simulink model "es6"  (Simulink 8.1)
settings: Solver=ode45  StartTime=0.0  StopTime=10  RelTol=1e-3
libraries: cstblocks x4
settings Model: Creator=nessuno  LastModifiedBy=paolo
settings DataIOCC: SignalLoggingSaveFormat=Dataset
settings OptimizationCC: ExpressionDepthLimit=128
settings DebuggingCC: FcnCallInpInsideContextMsg=EnableAllAsError
settings GRTTargetCC: CombineOutputUpdateFcns=on  GRTInterface=off

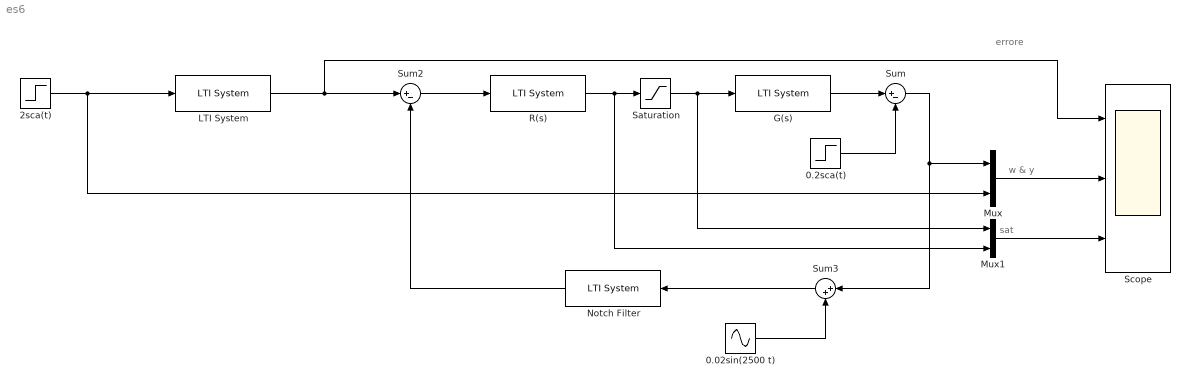
== system es6 ==
  note: sat
  note: w & y
  note: errore
  0.02sin(2500 t) : Sin  Amplitude=0.02  Frequency=2500  SampleTime=0
  0.2sca(t) : Step  Time=0  Before=1  After=0.2  SampleTime=0
  2sca(t) : Step  Time=2  After=2  SampleTime=0
  G(s) : cstblocks/LTI System  sys=G  IC=[]
  LTI System : cstblocks/LTI System  sys=PF  IC=[]
  Mux : Mux  Inputs=2
  Mux1 : Mux  Inputs=2
  Notch Filter : cstblocks/LTI System  sys=F_notch  IC=[]
  R(s) : cstblocks/LTI System  sys=R  IC=[]
  Saturation : Saturate  UpperLimit=2.39  LowerLimit=-0.24
  Scope : Scope  NumInputPorts=3
      settings: ShowLegends=on  TimeRange=10  YMin=-5~-5~-5  YMax=5~5~5
  Sum : Sum  Inputs=|+-
  Sum2 : Sum  Inputs=|+-
  Sum3 : Sum  Inputs=|++
  wires:
  Sum/1 -> Sum3/1, Mux/1
  LTI System/1 -> Sum2/1, Scope/1
  Sum2/1 -> R(s)/1
  G(s)/1 -> Sum/1
  R(s)/1 -> Mux1/2, Saturation/1
  Saturation/1 -> Mux1/1, G(s)/1
  0.2sca(t)/1 -> Sum/2
  0.02sin(2500 t)/1 -> Sum3/2
  Sum3/1 -> Notch Filter/1
  Notch Filter/1 -> Sum2/2
  2sca(t)/1 -> Mux/2, LTI System/1
  Mux/1 -> Scope/2
  Mux1/1 -> Scope/3
